simulink model "sim3d_visualization"  (R2024a)
settings: Solver=VariableStepAuto  StartTime=0  StopTime=20  FixedStep=timeStep  RelTol=1e-3
libraries: sim3dlib x4, sim3dautolib x1
settings Model: Creator=The MathWorks, Inc.  LastModifiedBy=nobuakif
settings DataIOCC: SaveOutput=off  DSMLogging=off  InspectSignalLogs=on  SaveTime=off  ReturnWorkspaceOutputs=off
settings OptimizationCC: DefaultParameterBehavior=Inlined  ReuseModelBlockBuffer=off
settings DebuggingCC: ParameterTunabilityLossMsg=error  UnconnectedInputMsg=warning  UnconnectedOutputMsg=warning  UnconnectedLineMsg=warning
settings ModelReferenceCC: EnableRefExpFcnMdlSchedulingChecks=on  PropagateSignalLabelsOutOfModel=off
settings RTWCC: GenCodeOnly=on  GenerateReport=on  GPUComputeCapability=3.5
settings CodeAppCC: ForceParamTrailComments=on
settings GRTTargetCC: TargetLangStandard=C89/C90 (ANSI)

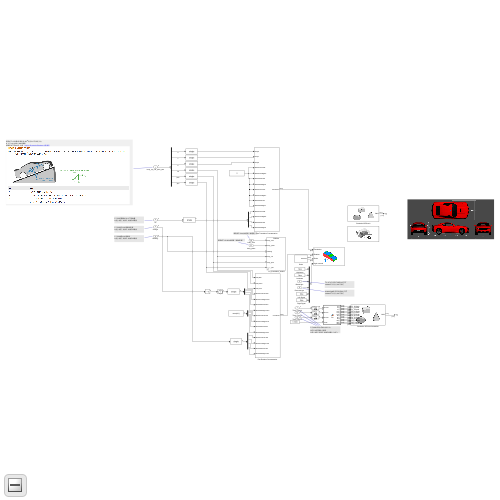
[thumbnail: Simulink's stored preview of the top-level diagram]
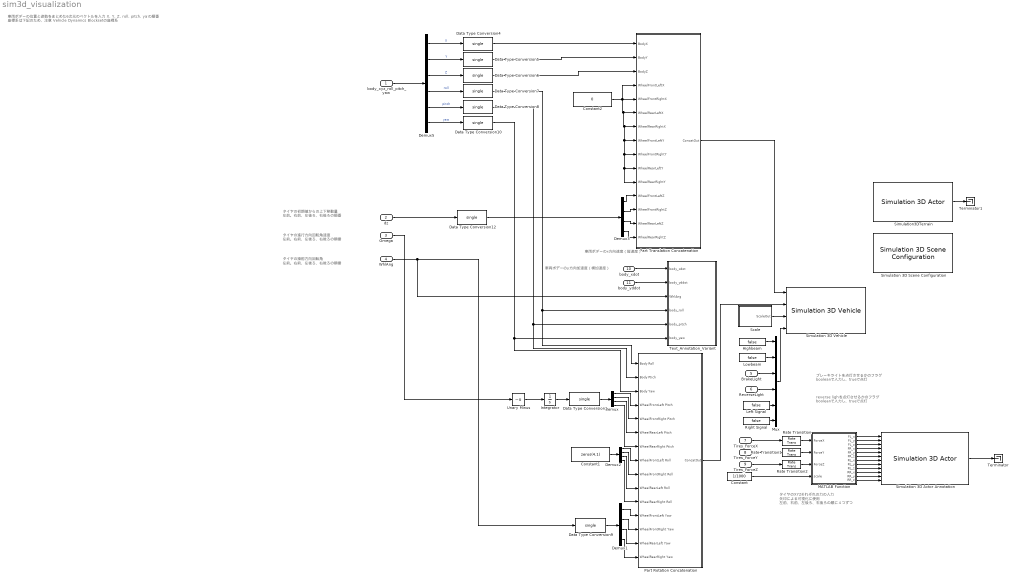
== system sim3d_visualization ==
  note: タイヤの初期値からの上下移動量
      | 左前。右前、左後ろ、右後ろの順番
  note: 車両ボデーの位置と姿勢をまとめた6次元のベクトルを入力
      | X, Y, Z, roll, pitch, yawの順番
      | 座標系は下記のため、注意 Vehicle Dynamics Blockset の座標系
  note: タイヤの進行方向回転角速度
      | 左前。右前、左後ろ、右後ろの順番
  note: タイヤの操舵方向回転角
      | 左前。右前、左後ろ、右後ろの順番
  note: ブレーキライトを点灯させるかのフラグ
      | booleanで入力し、trueで点灯
  note: reverse lightを点灯させるかのフラグ
      | booleanで入力し、trueで点灯
  note: 車両ボデーのx方向速度（縦速度）
  note: 車両ボデーのy方向加速度（横加速度）
  note: タイヤのXYZそれぞれの力の入力
      | 矢印による可視化に使用
      | 左前、右前、左後ろ、右後ろの順に４つずつ
  body_xyz_roll_pitch_yaw : Inport  OutDataTypeStr=single
  dz : Inport  Port=2  OutDataTypeStr=single
  Omega : Inport  Port=3  OutDataTypeStr=double
  WhlAng : Inport  Port=4  OutDataTypeStr=single
  BrakeLight : Inport  Port=5  OutDataTypeStr=boolean
  ReverseLight : Inport  Port=6  OutDataTypeStr=boolean
  Tires_ForceX : Inport  Port=7  OutDataTypeStr=single  PortDimensions=4
  Tires_ForceY : Inport  Port=8  OutDataTypeStr=single  PortDimensions=4
  Tires_ForceZ : Inport  Port=9  OutDataTypeStr=single  PortDimensions=4
  body_xdot : Inport  Port=10  OutDataTypeStr=single
  body_yddot : Inport  Port=11  OutDataTypeStr=single
  Constant : Constant  Value=1/1000
  Constant1 : Constant  Value=zeros(4,1)  OutDataTypeStr=single
  Constant2 : Constant  Value=0  OutDataTypeStr=single
  Data Type Conversion{1,4..10,12} (9 alike) : DataTypeConversion  OutDataTypeStr=single  SaturateOnIntegerOverflow=off  RndMeth=Floor
  Demux{,1..3} (4 alike) : Demux
  Demux5 : Demux  Outputs=6
  Highbeam : Constant  Value=false
  Integrator : Integrator  WrapState=on  WrappedStateUpperValue=2*pi  WrappedStateLowerValue=0  ZeroCross=off
  Left Signal : Constant  Value=false
  Lowbeam : Constant  Value=false
  MATLAB Function : MATLAB Function  TreatAsAtomicUnit=on
  Mux : Mux  Inputs=6
  Part Rotation Concatenation : Subsystem
  Part Translation Concatenation : Subsystem
  Rate Transition : RateTransition  OutPortSampleTime=0.1
  Rate Transition1 : RateTransition  OutPortSampleTime=0.1
  Rate Transition2 : RateTransition  OutPortSampleTime=0.1
  Right Signal : Constant  Value=false
  Scale : Subsystem
  Simulation 3D Actor Annotation : sim3dlib/Simulation 3D Actor  Priority=1  ActorName=Sim3dActor_annotation  ParentName=SimulinkVehicle1  Operation=Create at setup  InitScriptText=|  SampleTime=-1  Translation=single([0 0 0])  Rotation=single([0 0 0])  Scale=single([1 1 1])  InputsText=|  aMode=5  ActorTag=Sim3dActor_annotation  ActorType=Sim3dActor  ID=C
      InitScriptText=|
      | y_offset = 1; z_offset = 0.1;
      | fl_pos = [1.491, 1.713/2+y_offset, z_offset];
      | fr_pos = [1.491, -1.713/2-y_offset, z_offset];
      | rl_pos = [-1.592, 1.713/2+y_offset, z_offset];
      | rr_pos = [-1.592, -1.713/2-y_offset, z_offset];
      | 
      | arrowfl = sim3d.graphics.Arrow("ActorName", "FL_Z");
      | arrowfl.CoordinateSystem = "MATLAB";
      | arrowfl.Color = [0, 0, 1];
      | arrowfl.Rotation = [0, -pi/2, 0];
      | arrowfl.Scale = [1, 1, 1]*2;
      | World.add(arrowfl, Actor);
      | arrowfl.Translation = fl_pos;
      | 
      | arrowfl_x = sim3d.graphics.Arrow("ActorName", "FL_X");
      | arrowfl_x.CoordinateSystem = "MATLAB";
      | arrowfl_x.Color = [1, 0, 0];
      | arrowfl_x.Rotation = [0, 0, 0];
      | arrowfl_x.Scale = [1, 1, 1]*2;
      | World.add(arrowfl_x, Actor);
      | arrowfl_x.Translation = fl_pos;
      | 
      | arrowfl_y = sim3d.graphics.Arrow("ActorName", "FL_Y");
      | arrowfl_y.CoordinateSystem = "MATLAB";
      | arrowfl_y.Color = [0, 1, 0];
      | arrowfl_y.Rotation = [0, 0, pi/2];
      | arrowfl_y.Scale = [1, 1, 1]*2;
      | World.add(arrowfl_y, Actor);
      | arrowfl_y.Translation = fl_pos;
      | 
      | 
      | arrowfr = sim3d.graphics.Arrow("ActorName", "FR_Z");
      | arrowfr.CoordinateSystem = "MATLAB";
      | arrowfr.Color = [0, 0, 1];
      | arrowfr.Rotation = [0, -pi/2, 0];
      | arrowfr.Scale = [1, 1, 1] * 2;
      | World.add(arrowfr, Actor);
      | arrowfr.Translation = fr_pos;
      | 
      | arrowfr_x = sim3d.graphics.Arrow("ActorName", "FR_X");
      | arrowfr_x.CoordinateSystem = "MATLAB";
      | arrowfr_x.Color = [1, 0, 0];
      | arrowfr_x.Rotation = [0, 0, 0];
      | arrowfr_x.Scale = [1, 1, 1]*2;
      | World.add(arrowfr_x, Actor);
      | arrowfr_x.Translation = fr_pos;
      | 
      | arrowfr_y = sim3d.graphics.Arrow("ActorName", "FR_Y");
      | arrowfr_y.CoordinateSystem = "MATLAB";
      | arrowfr_y.Color = [0, 1, 0];
      | arrowfr_y.Rotation = [0, 0, pi/2];
      | arrowfr_y.Scale = [1, 1, 1]*2;
      | World.add(arrowfr_y, Actor);
      | arrowfr_y.Translation = fr_pos;
      | 
      | 
      | arrowrl = sim3d.graphics.Arrow("ActorName", "RL_Z");
      | arrowrl.CoordinateSystem = "MATLAB";
      | arrowrl.Color = [0, 0, 1];
      | arrowrl.Rotation = [0, -pi/2, 0];
      | arrowrl.Scale = [1, 1, 1] * 2;
      | World.add(arrowrl, Actor);
      | arrowrl.Translation = rl_pos;
      | 
      | arrowrl_x = sim3d.graphics.Arrow("ActorName", "RL_X");
      | arrowrl_x.CoordinateSystem = "MATLAB";
      | arrowrl_x.Color = [1, 0, 0];
      | arrowrl_x.Rotation = [0, 0, 0];
      | arrowrl_x.Scale = [1, 1, 1]*2;
      | World.add(arrowrl_x, Actor);
      | arrowrl_x.Translation = rl_pos;
      | 
      | arrowrl_y = sim3d.graphics.Arrow("ActorName", "RL_Y");
      | arrowrl_y.CoordinateSystem = "MATLAB";
      | arrowrl_y.Color = [0, 1, 0];
      | arrowrl_y.Rotation = [0, 0, pi/2];
      | arrowrl_y.Scale = [1, 1, 1]*2;
      | World.add(arrowrl_y, Actor);
      | arrowrl_y.Translation = rl_pos;
      | 
      | 
      | arrowrr = sim3d.graphics.Arrow("ActorName", "RR_Z");
      | arrowrr.CoordinateSystem = "MATLAB";
      | arrowrr.Color = [0, 0, 1];
      | arrowrr.Rotation = [0, -pi/2, 0];
      | arrowrr.Scale = [1, 1, 1]*2;
      | World.add(arrowrr, Actor);
      | arrowrr.Translation = rr_pos;
      | 
      | arrowrr_x = sim3d.graphics.Arrow("ActorName", "RR_X");
      | arrowrr_x.CoordinateSystem = "MATLAB";
      | arrowrr_x.Color = [1, 0, 0];
      | arrowrr_x.Rotation = [0, 0, 0];
      | arrowrr_x.Scale = [1, 1, 1]*2;
      | World.add(arrowrr_x, Actor);
      | arrowrr_x.Translation = rr_pos;
      | 
      | arrowrr_y = sim3d.graphics.Arrow("ActorName", "RR_Y");
      | arrowrr_y.CoordinateSystem = "MATLAB";
      | arrowrr_y.Color = [0, 1, 0];
      | arrowrr_y.Rotation = [0, 0, pi/2];
      | arrowrr_y.Scale = [1, 1, 1]*2;
      | World.add(arrowrr_y, Actor);
      | arrowrr_y.Translation = rr_pos;
      InputsText=|
      | FL_X.Scale
      | FL_Y.Scale
      | FL_Z.Scale
      | FR_X.Scale
      | FR_Y.Scale
      | FR_Z.Scale
      | RL_X.Scale
      | RL_Y.Scale
      | RL_Z.Scale
      | RR_X.Scale
      | RR_Y.Scale
      | RR_Z.Scale
  Simulation 3D Scene Configuration : sim3dlib/Simulation 3D Scene Configuration  Priority=0  ProjectFormat=Default Scenes  SceneDesc=Empty scene  ProjectName=D:\MATLAB\R2024a\toolbox\shared\sim3d_projects\automotive_project_windows\UE\WindowsNoEditor\VehicleSimulation.exe  ScenePath=/Game/Maps/HwStrght  RoadRunnerProjectPath=D:\MATLAB\RoadRunnerSimulinkHandson_github\CRG\crgRoad.stl  EnableOpenDRIVE=off  vehTagList={'Custom';'Scene Origin';'Sim3dActor1';'Sim3dActor_annotation';'Sim3dActor_text';'SimulinkVehicle1'}  vehTag=SimulinkVehicle1  FreeCameraInitialTranslation=[0, 0, 0]  FreeCameraDefaultInitialTranslation=[-6, 0, 2]  FreeCameraInitialRotation=[0, 0, 0]  FreeCameraDefaultInitialRotation=[0, -15, 0]  OpVisEn=off  Ts=0.1  EnableWindow=on  EnableRemoteAccess=off  EnableWeather=off  SunAzimuth=90  SunAltitude=40.0  EnableGeospatialSun=off  Latitude=0  Longitude=0  Date=2023-01-01  Time=10:30:00  GeoTimeZone=-5.0  SunDaylightSaving=off  wind=1  clouds=10  EnableVolumetricClouds=off  CloudCoverage=0  CloudAltitude=6  fog=0  rain=0  RaindropsEffect=off  SnowDensity=0  EnableGeospatial=off  UseTrueOrigin=off  OriginHeight=200  OriginLatitude=40.744652  OriginLongitude=-73.988864  MapStyle=Aerial  AdditionalAssetIDs=[]  UseAdvancedSunSky=off  SolarTime=11  TimeZone=-5  Day=21  Month=9  Year=2022  UseDaylightSavingTime=on  DSTStartDay=10  DSTStartMonth=3  DSTEndDay=3  DSTEndMonth=11  DSTSwitchHour=2  sensorTag=MainCamera1  sensorId=1  sensorName=MainCamera1  mountLoc=Origin  offsetFlag=off  tmountOffset=[0, 0, 0]  rmountOffset=[0, 0, 0]  HorizontalResolution=1280  VerticalResolution=720  HorizontalFOV=60  mountPoint=[0 0 0]  mountOrientation=[0 0 0]  aMode=5  ID=1  GeoTrigger=Inactive
      settings: LibrarySourceBlock=sl3dlib/Simulation 3D/Simulation 3D Scene Configuration
  Simulation 3D Vehicle : sim3dautolib/Simulation 3D Vehicle  Priority=-1  PassVehMesh=Muscle car  MeshPath=/MathWorksSimulation/Vehicles/Muscle/Meshes/SK_MuscleCar.SK_MuscleCar  VehColor=Red  ActorName=SimulinkVehicle1  VehLightsControl=on  HeadlightColor=[ 1, 1, 1 ]  HighBeamIntensity=100000  LowBeamIntensity=60000  HighBeamConeAngle=1.22  LowBeamConeAngle=1.22  LeftHeadlightOrientation=[ 0, 0 ]  RightHeadlightOrientation=[ 0, 0 ]  BrakelightIntensity=500  ReverselightIntensity=500  SignallightIntensity=500  SignallightPeriod=1  SignalPulseWidth=50  Translation=zeros(5,3)  Rotation=zeros(5,3)  Scale=ones( 5, 3 )  SampleTime=-1  ActorType=SimulinkVehicle  ID=1  aMode=2  ActorTag=SimulinkVehicle1
  Simulation3DTerrain : sim3dlib/Simulation 3D Actor  Priority=1  ActorName=Sim3dActor1  ParentName=Scene Origin  Operation=Create at setup  InitScriptText="Actor.CoordinateSystem = \"MATLAB\";"  SampleTime=-1  Translation=[0 0 0]  Rotation=[0 0 0]  Scale=[1 1 1]  aMode=5  ActorTag=Sim3dActor1  ActorType=Sim3dActor  ID=1
  Terminator : Terminator
  Terminator1 : Terminator
  Text_Annotation_Variant : Subsystem  Priority=1  Variant=on
  Unary Minus : UnaryMinus
  wires:
  Demux5/6 -> Data Type Conversion10/1  "yaw"
  Demux5/3 -> Data Type Conversion6/1  "Z"
  MATLAB Function/5(FR_y) -> Simulation 3D Actor Annotation/5
  MATLAB Function/8(RL_y) -> Simulation 3D Actor Annotation/8
  Right Signal/1 -> Mux/6
  Demux3/2 -> Part Translation Concatenation/13(WheelFrontRightZ)
  MATLAB Function/9(RL_z) -> Simulation 3D Actor Annotation/9
  Mux/1 -> Simulation 3D Vehicle/4
  Constant1/1 -> Demux2/1
  Data Type Conversion6/1 -> Part Translation Concatenation/3(BodyZ)
  MATLAB Function/1(FL_x) -> Simulation 3D Actor Annotation/1
  Omega/1 -> Unary Minus/1
  Part Translation Concatenation/1(ConcatOut) -> Simulation 3D Vehicle/1
  MATLAB Function/11(RR_y) -> Simulation 3D Actor Annotation/11
  MATLAB Function/7(RL_x) -> Simulation 3D Actor Annotation/7
  Demux3/3 -> Part Translation Concatenation/14(WheelRearLeftZ)
  Demux5/4 -> Data Type Conversion7/1  "roll"
  MATLAB Function/2(FL_y) -> Simulation 3D Actor Annotation/2
  Demux1/2 -> Part Rotation Concatenation/13(WheelFrontRight Yaw)
  Demux3/1 -> Part Translation Concatenation/12(WheelFrontLeftZ)
  Demux2/1 -> Part Rotation Concatenation/8(WheelFrontLeft Roll)
  Demux2/3 -> Part Rotation Concatenation/10(WheelRearLeft Roll)
  Tires_ForceY/1 -> Rate Transition1/1
  Tires_ForceX/1 -> Rate Transition/1
  Unary Minus/1 -> Integrator/1
  Lowbeam/1 -> Mux/2
  MATLAB Function/6(FR_z) -> Simulation 3D Actor Annotation/6
  MATLAB Function/10(RR_x) -> Simulation 3D Actor Annotation/10
  MATLAB Function/4(FR_x) -> Simulation 3D Actor Annotation/4
  Constant2/1 -> Part Translation Concatenation/5(WheelFrontRightX), Part Translation Concatenation/6(WheelRearLeftX), Part Translation Concatenation/7(WheelRearRightX), Part Translation Concatenation/8(WheelFrontLeftY), Part Translation Concatenation/9(WheelFrontRightY), Part Translation Concatenation/10(WheelRearLeftY), Part Translation Concatenation/11(WheelRearRightY), Part Translation Concatenation/4(WheelFrontLeftX)
  BrakeLight/1 -> Mux/3
  Part Rotation Concatenation/1(ConcatOut) -> Simulation 3D Vehicle/2
  Data Type Conversion7/1 -> Text_Annotation_Variant/4(body_roll), Part Rotation Concatenation/1(Body Roll)
  MATLAB Function/3(FL_z) -> Simulation 3D Actor Annotation/3
  Integrator/1 -> Data Type Conversion1/1
  Demux5/5 -> Data Type Conversion8/1  "pitch"
  Simulation 3D Actor Annotation/1 -> Terminator/1
  Data Type Conversion4/1 -> Part Translation Concatenation/1(BodyX)
  Left Signal/1 -> Mux/5
  Demux5/1 -> Data Type Conversion4/1  "X"
  Demux/3 -> Part Rotation Concatenation/6(WheelRearLeft Pitch)
  Demux5/2 -> Data Type Conversion5/1  "Y"
  Data Type Conversion12/1 -> Demux3/1
  Demux1/4 -> Part Rotation Concatenation/15(WheelRearRight Yaw)
  Data Type Conversion8/1 -> Part Rotation Concatenation/2(Body Ptich), Text_Annotation_Variant/5(body_pitch)
  ReverseLight/1 -> Mux/4
  Demux1/1 -> Part Rotation Concatenation/12(WheelFrontLeft Yaw)
  Tires_ForceZ/1 -> Rate Transition2/1
  Data Type Conversion9/1 -> Demux1/1
  MATLAB Function/12(RR_z) -> Simulation 3D Actor Annotation/12
  Data Type Conversion10/1 -> Part Rotation Concatenation/3(Body Yaw), Text_Annotation_Variant/6(body_yaw)
  Scale/1(ScaleOut) -> Simulation 3D Vehicle/3
  Demux/1 -> Part Rotation Concatenation/4(WheelFrontLeft Pitch)
  Highbeam/1 -> Mux/1
  Demux3/4 -> Part Translation Concatenation/15(WheelRearRightZ)
  WhlAng/1 -> Text_Annotation_Variant/3(WhlAng), Data Type Conversion9/1
  dz/1 -> Data Type Conversion12/1
  Demux/2 -> Part Rotation Concatenation/5(WheelFrontRight Pitch)
  Demux2/4 -> Part Rotation Concatenation/11(WheelRearRight Roll)
  Demux2/2 -> Part Rotation Concatenation/9(WheelFrontRight Roll)
  Data Type Conversion5/1 -> Part Translation Concatenation/2(BodyY)
  Demux/4 -> Part Rotation Concatenation/7(WheelRearRight Ptich)
  Demux1/3 -> Part Rotation Concatenation/14(WheelRearLeft Yaw)
  body_xyz_roll_pitch_yaw/1 -> Demux5/1
  body_xdot/1 -> Text_Annotation_Variant/1(body_xdot)
  body_yddot/1 -> Text_Annotation_Variant/2(body_yddot)
  Constant/1 -> MATLAB Function/4(scale)
  Data Type Conversion1/1 -> Demux/1
  Simulation3DTerrain/1 -> Terminator1/1
  Rate Transition/1 -> MATLAB Function/1(ForceX)
  Rate Transition1/1 -> MATLAB Function/2(ForceY)
  Rate Transition2/1 -> MATLAB Function/3(ForceZ)

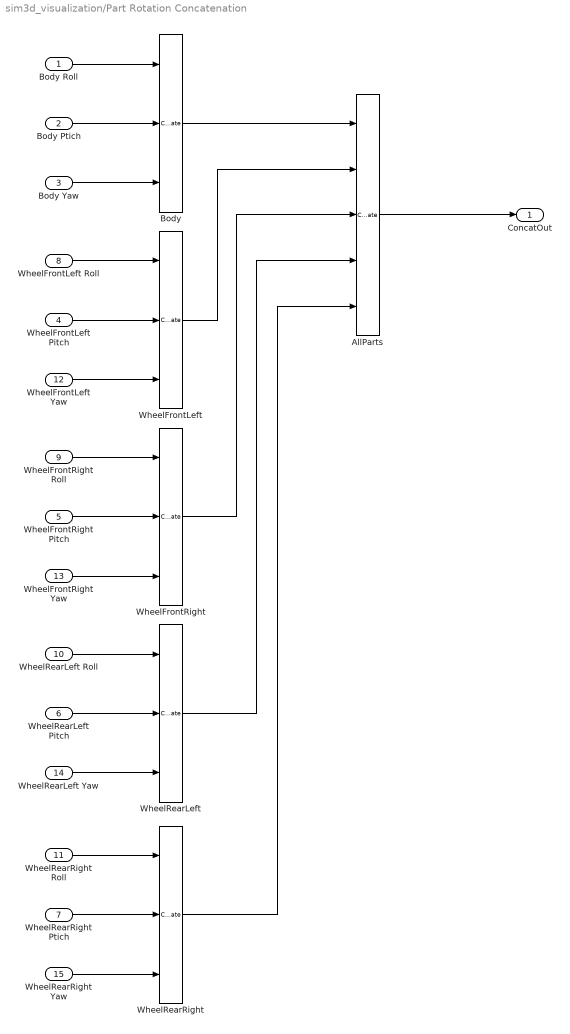
== system sim3d_visualization/Part Rotation Concatenation ==
  Body Roll : Inport
  Body Ptich : Inport  Port=2
  Body Yaw : Inport  Port=3
  WheelFrontLeft Pitch : Inport  Port=4
  WheelFrontRight Pitch : Inport  Port=5
  WheelRearLeft Pitch : Inport  Port=6
  WheelRearRight Ptich : Inport  Port=7
  WheelFrontLeft Roll : Inport  Port=8
  WheelFrontRight Roll : Inport  Port=9
  WheelRearLeft Roll : Inport  Port=10
  WheelRearRight Roll : Inport  Port=11
  WheelFrontLeft Yaw : Inport  Port=12
  WheelFrontRight Yaw : Inport  Port=13
  WheelRearLeft Yaw : Inport  Port=14
  WheelRearRight Yaw : Inport  Port=15
  AllParts : Concatenate  NumInputs=5  Mode=Multidimensional array
  Body : Concatenate  NumInputs=3  Mode=Multidimensional array  ConcatenateDimension=2
  WheelFrontLeft : Concatenate  NumInputs=3  Mode=Multidimensional array  ConcatenateDimension=2
  WheelFrontRight : Concatenate  NumInputs=3  Mode=Multidimensional array  ConcatenateDimension=2
  WheelRearLeft : Concatenate  NumInputs=3  Mode=Multidimensional array  ConcatenateDimension=2
  WheelRearRight : Concatenate  NumInputs=3  Mode=Multidimensional array  ConcatenateDimension=2
  ConcatOut : Outport  VectorParamsAs1DForOutWhenUnconnected=off
  wires:
  Body Yaw/1 -> Body/3
  WheelFrontLeft Yaw/1 -> WheelFrontLeft/3
  WheelFrontLeft/1 -> AllParts/2
  Body/1 -> AllParts/1
  WheelRearLeft/1 -> AllParts/4
  WheelFrontRight/1 -> AllParts/3
  WheelRearRight Yaw/1 -> WheelRearRight/3
  WheelRearLeft Yaw/1 -> WheelRearLeft/3
  AllParts/1 -> ConcatOut/1
  WheelRearRight/1 -> AllParts/5
  WheelFrontRight Yaw/1 -> WheelFrontRight/3
  Body Roll/1 -> Body/1
  Body Ptich/1 -> Body/2
  WheelFrontLeft Pitch/1 -> WheelFrontLeft/2
  WheelFrontLeft Roll/1 -> WheelFrontLeft/1
  WheelFrontRight Roll/1 -> WheelFrontRight/1
  WheelFrontRight Pitch/1 -> WheelFrontRight/2
  WheelRearLeft Roll/1 -> WheelRearLeft/1
  WheelRearLeft Pitch/1 -> WheelRearLeft/2
  WheelRearRight Roll/1 -> WheelRearRight/1
  WheelRearRight Ptich/1 -> WheelRearRight/2

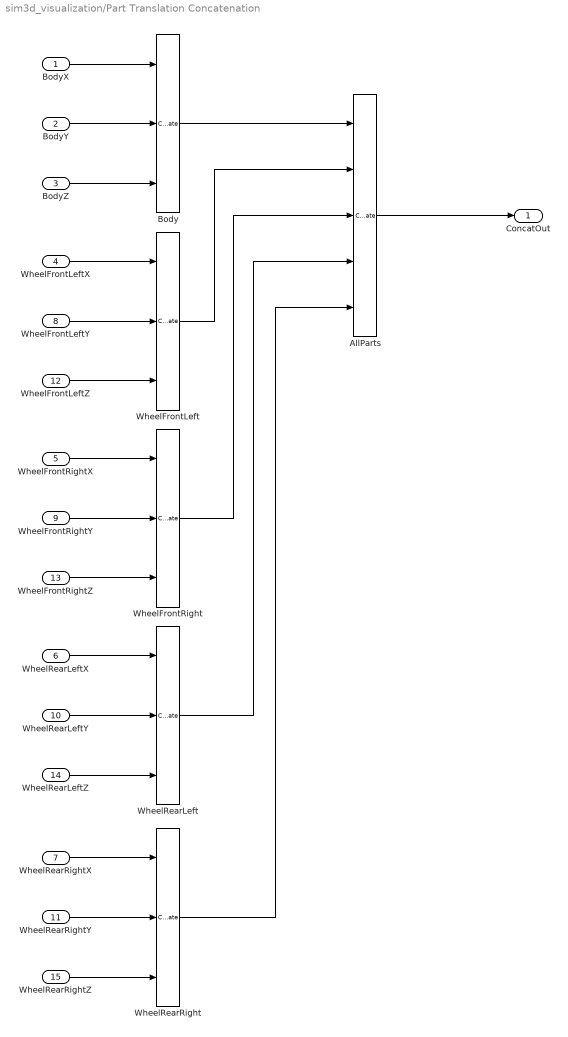
== system sim3d_visualization/Part Translation Concatenation ==
  BodyX : Inport
  BodyY : Inport  Port=2
  BodyZ : Inport  Port=3
  WheelFrontLeftX : Inport  Port=4
  WheelFrontRightX : Inport  Port=5
  WheelRearLeftX : Inport  Port=6
  WheelRearRightX : Inport  Port=7
  WheelFrontLeftY : Inport  Port=8
  WheelFrontRightY : Inport  Port=9
  WheelRearLeftY : Inport  Port=10
  WheelRearRightY : Inport  Port=11
  WheelFrontLeftZ : Inport  Port=12
  WheelFrontRightZ : Inport  Port=13
  WheelRearLeftZ : Inport  Port=14
  WheelRearRightZ : Inport  Port=15
  AllParts : Concatenate  NumInputs=5  Mode=Multidimensional array
  Body : Concatenate  NumInputs=3  Mode=Multidimensional array  ConcatenateDimension=2
  WheelFrontLeft : Concatenate  NumInputs=3  Mode=Multidimensional array  ConcatenateDimension=2
  WheelFrontRight : Concatenate  NumInputs=3  Mode=Multidimensional array  ConcatenateDimension=2
  WheelRearLeft : Concatenate  NumInputs=3  Mode=Multidimensional array  ConcatenateDimension=2
  WheelRearRight : Concatenate  NumInputs=3  Mode=Multidimensional array  ConcatenateDimension=2
  ConcatOut : Outport  VectorParamsAs1DForOutWhenUnconnected=off
  wires:
  BodyX/1 -> Body/1
  BodyZ/1 -> Body/3
  WheelFrontLeftX/1 -> WheelFrontLeft/1
  WheelFrontLeftZ/1 -> WheelFrontLeft/3
  WheelFrontLeftY/1 -> WheelFrontLeft/2
  BodyY/1 -> Body/2
  WheelFrontLeft/1 -> AllParts/2
  WheelRearRightX/1 -> WheelRearRight/1
  Body/1 -> AllParts/1
  WheelRearLeft/1 -> AllParts/4
  WheelFrontRight/1 -> AllParts/3
  WheelRearRightZ/1 -> WheelRearRight/3
  WheelFrontRightY/1 -> WheelFrontRight/2
  WheelFrontRightX/1 -> WheelFrontRight/1
  WheelRearRightY/1 -> WheelRearRight/2
  WheelRearLeftZ/1 -> WheelRearLeft/3
  AllParts/1 -> ConcatOut/1
  WheelRearLeftY/1 -> WheelRearLeft/2
  WheelRearRight/1 -> AllParts/5
  WheelRearLeftX/1 -> WheelRearLeft/1
  WheelFrontRightZ/1 -> WheelFrontRight/3

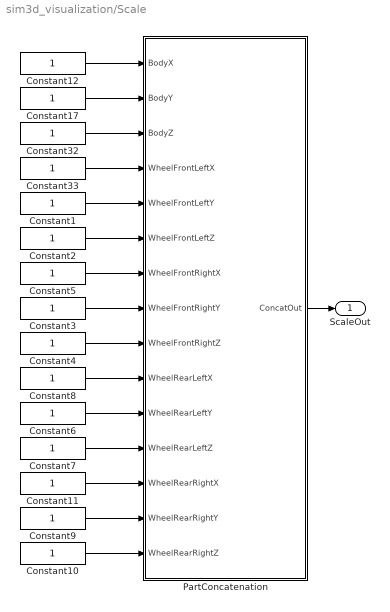
== system sim3d_visualization/Scale ==
  Constant{1..12,17,32..33} (15 alike) : Constant  OutDataTypeStr=single
  PartConcatenation : Subsystem
  ScaleOut : Outport  VectorParamsAs1DForOutWhenUnconnected=off
  wires:
  Constant10/1 -> PartConcatenation/15(WheelRearRightZ)
  Constant9/1 -> PartConcatenation/14(WheelRearRightY)
  Constant11/1 -> PartConcatenation/13(WheelRearRightX)
  Constant7/1 -> PartConcatenation/12(WheelRearLeftZ)
  Constant6/1 -> PartConcatenation/11(WheelRearLeftY)
  Constant8/1 -> PartConcatenation/10(WheelRearLeftX)
  Constant4/1 -> PartConcatenation/9(WheelFrontRightZ)
  Constant3/1 -> PartConcatenation/8(WheelFrontRightY)
  Constant5/1 -> PartConcatenation/7(WheelFrontRightX)
  Constant2/1 -> PartConcatenation/6(WheelFrontLeftZ)
  Constant1/1 -> PartConcatenation/5(WheelFrontLeftY)
  Constant33/1 -> PartConcatenation/4(WheelFrontLeftX)
  Constant32/1 -> PartConcatenation/3(BodyZ)
  Constant17/1 -> PartConcatenation/2(BodyY)
  Constant12/1 -> PartConcatenation/1(BodyX)
  PartConcatenation/1(ConcatOut) -> ScaleOut/1

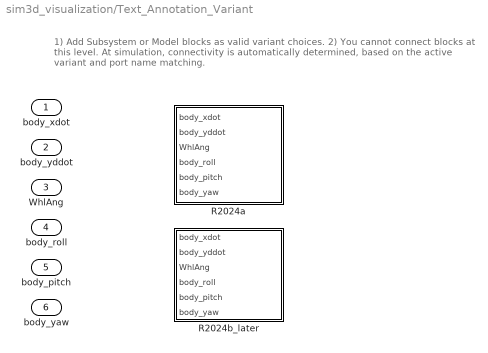
== system sim3d_visualization/Text_Annotation_Variant ==
  note: 1) Add Subsystem or Model blocks as valid variant choices.
      | 2) You cannot connect blocks at this level. At simulation, connectivity is automatically
      | determined, based on the active variant and port name matching.
  body_xdot : Inport
  body_yddot : Inport  Port=2
  WhlAng : Inport  Port=3
  body_roll : Inport  Port=4
  body_pitch : Inport  Port=5
  body_yaw : Inport  Port=6
  R2024a : Subsystem  VariantControl=str2num(ver('simulink').Version) <= 24.1
  R2024b_later : Subsystem  VariantControl=str2num(ver('simulink').Version) > 24.1

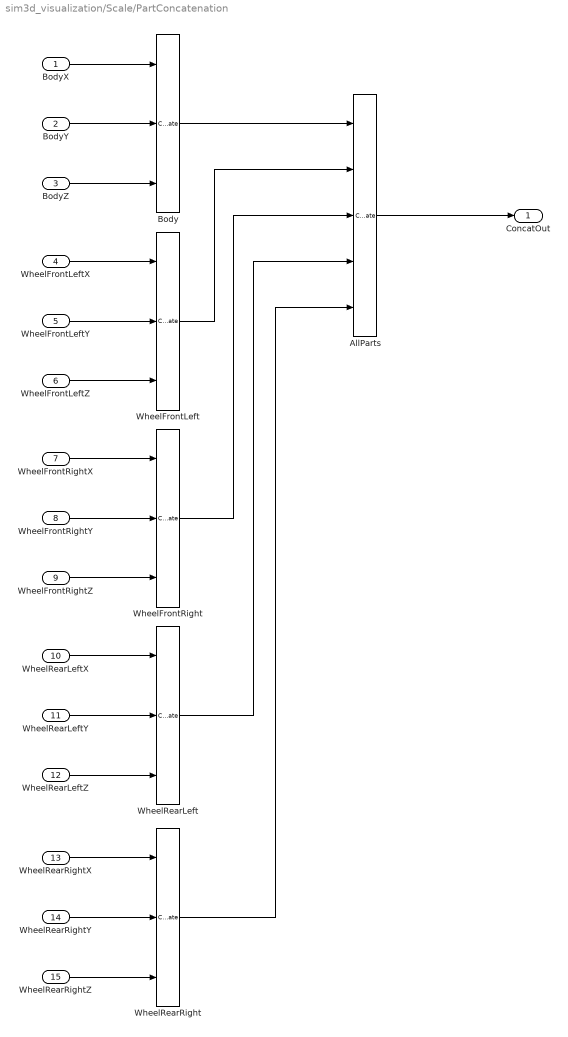
== system sim3d_visualization/Scale/PartConcatenation ==
  BodyX : Inport
  BodyY : Inport  Port=2
  BodyZ : Inport  Port=3
  WheelFrontLeftX : Inport  Port=4
  WheelFrontLeftY : Inport  Port=5
  WheelFrontLeftZ : Inport  Port=6
  WheelFrontRightX : Inport  Port=7
  WheelFrontRightY : Inport  Port=8
  WheelFrontRightZ : Inport  Port=9
  WheelRearLeftX : Inport  Port=10
  WheelRearLeftY : Inport  Port=11
  WheelRearLeftZ : Inport  Port=12
  WheelRearRightX : Inport  Port=13
  WheelRearRightY : Inport  Port=14
  WheelRearRightZ : Inport  Port=15
  AllParts : Concatenate  NumInputs=5  Mode=Multidimensional array
  Body : Concatenate  NumInputs=3  Mode=Multidimensional array  ConcatenateDimension=2
  WheelFrontLeft : Concatenate  NumInputs=3  Mode=Multidimensional array  ConcatenateDimension=2
  WheelFrontRight : Concatenate  NumInputs=3  Mode=Multidimensional array  ConcatenateDimension=2
  WheelRearLeft : Concatenate  NumInputs=3  Mode=Multidimensional array  ConcatenateDimension=2
  WheelRearRight : Concatenate  NumInputs=3  Mode=Multidimensional array  ConcatenateDimension=2
  ConcatOut : Outport  VectorParamsAs1DForOutWhenUnconnected=off
  wires:
  BodyX/1 -> Body/1
  BodyZ/1 -> Body/3
  WheelFrontLeftX/1 -> WheelFrontLeft/1
  WheelFrontLeftZ/1 -> WheelFrontLeft/3
  WheelFrontLeftY/1 -> WheelFrontLeft/2
  BodyY/1 -> Body/2
  WheelFrontLeft/1 -> AllParts/2
  WheelRearRightX/1 -> WheelRearRight/1
  Body/1 -> AllParts/1
  WheelRearLeft/1 -> AllParts/4
  WheelFrontRight/1 -> AllParts/3
  WheelRearRightZ/1 -> WheelRearRight/3
  WheelFrontRightY/1 -> WheelFrontRight/2
  WheelFrontRightX/1 -> WheelFrontRight/1
  WheelRearRightY/1 -> WheelRearRight/2
  WheelRearLeftZ/1 -> WheelRearLeft/3
  AllParts/1 -> ConcatOut/1
  WheelRearLeftY/1 -> WheelRearLeft/2
  WheelRearRight/1 -> AllParts/5
  WheelRearLeftX/1 -> WheelRearLeft/1
  WheelFrontRightZ/1 -> WheelFrontRight/3

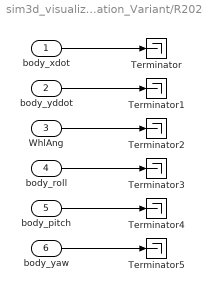
== system sim3d_visualization/Text_Annotation_Variant/R2024a ==
  body_xdot : Inport
  body_yddot : Inport  Port=2
  WhlAng : Inport  Port=3
  body_roll : Inport  Port=4
  body_pitch : Inport  Port=5
  body_yaw : Inport  Port=6
  Terminator{,1..5} (6 alike) : Terminator
  wires:
  body_xdot/1 -> Terminator/1
  body_yddot/1 -> Terminator1/1
  WhlAng/1 -> Terminator2/1
  body_roll/1 -> Terminator3/1
  body_pitch/1 -> Terminator4/1
  body_yaw/1 -> Terminator5/1

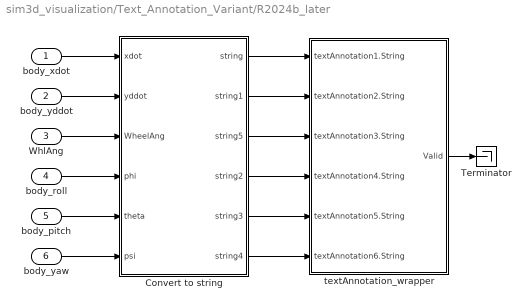
== system sim3d_visualization/Text_Annotation_Variant/R2024b_later ==
  body_xdot : Inport
  body_yddot : Inport  Port=2
  WhlAng : Inport  Port=3
  body_roll : Inport  Port=4
  body_pitch : Inport  Port=5
  body_yaw : Inport  Port=6
  Convert to string : Subsystem
  Terminator : Terminator
  textAnnotation_wrapper : Subsystem  Priority=1  Variant=on  AllowZeroVariantControls=on
  wires:
  Convert to string/5(string3) -> textAnnotation_wrapper/5(textAnnotation5.String)
  Convert to string/2(string1) -> textAnnotation_wrapper/2(textAnnotation2.String)
  Convert to string/4(string2) -> textAnnotation_wrapper/4(textAnnotation4.String)
  Convert to string/6(string4) -> textAnnotation_wrapper/6(textAnnotation6.String)
  Convert to string/3(string5) -> textAnnotation_wrapper/3(textAnnotation3.String)
  body_pitch/1 -> Convert to string/5(theta)
  body_yaw/1 -> Convert to string/6(psi)
  WhlAng/1 -> Convert to string/3(WheelAng)
  body_yddot/1 -> Convert to string/2(yddot)
  body_roll/1 -> Convert to string/4(phi)
  body_xdot/1 -> Convert to string/1(xdot)
  Convert to string/1(string) -> textAnnotation_wrapper/1(textAnnotation1.String)
  textAnnotation_wrapper/1(Valid) -> Terminator/1

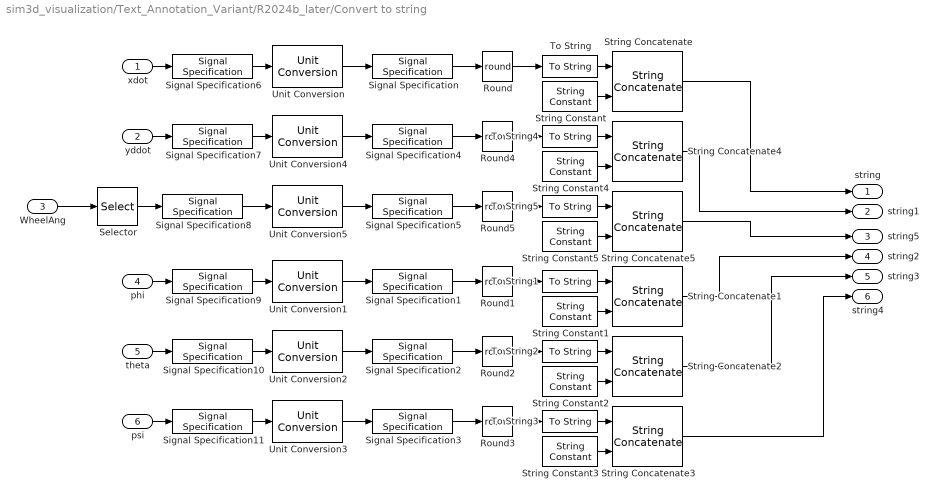
== system sim3d_visualization/Text_Annotation_Variant/R2024b_later/Convert to string ==
  xdot : Inport
  yddot : Inport  Port=2
  WheelAng : Inport  Port=3
  phi : Inport  Port=4
  theta : Inport  Port=5
  psi : Inport  Port=6
  Round{,1..5} (6 alike) : Rounding  Operator=round
  Selector : Selector  InputPortWidth=4  IndexOptions=Index vector (dialog)  Indices=[1]  OutputSizes=1
  Signal Specification : SignalSpecification  Unit=km/h
  Signal Specification{1..3,5} (4 alike) : SignalSpecification  Unit=deg
  Signal Specification{8..11} (4 alike) : SignalSpecification  Unit=rad
  Signal Specification4 : SignalSpecification  Unit=m/s^2
  Signal Specification6 : SignalSpecification  Unit=m/s
  Signal Specification7 : SignalSpecification  Unit=m/s^2
  String Concatenate{,1..5} (6 alike) : StringConcatenate
  String Constant : StringConstant  String="\" km/h\""
  String Constant{1..3,5} (4 alike) : StringConstant  String="\" deg\""
  String Constant4 : StringConstant  String="\" m/s^2\""
  To String{,1..5} (6 alike) : ToString
  Unit Conversion{,1..5} (6 alike) : UnitConversion
  string : Outport
  string1 : Outport  Port=2
  string5 : Outport  Port=3
  string2 : Outport  Port=4
  string3 : Outport  Port=5
  string4 : Outport  Port=6
  wires:
  Selector/1 -> Signal Specification8/1
  String Concatenate5/1 -> string5/1
  WheelAng/1 -> Selector/1
  String Constant5/1 -> String Concatenate5/2
  To String5/1 -> String Concatenate5/1
  Signal Specification5/1 -> Round5/1
  Round5/1 -> To String5/1
  Unit Conversion5/1 -> Signal Specification5/1
  String Concatenate4/1 -> string1/1
  yddot/1 -> Signal Specification7/1
  Unit Conversion4/1 -> Signal Specification4/1
  Round4/1 -> To String4/1
  Signal Specification4/1 -> Round4/1
  To String4/1 -> String Concatenate4/1
  String Constant4/1 -> String Concatenate4/2
  String Concatenate3/1 -> string4/1
  String Concatenate2/1 -> string3/1
  String Concatenate1/1 -> string2/1
  String Concatenate/1 -> string/1
  theta/1 -> Signal Specification10/1
  psi/1 -> Signal Specification11/1
  Unit Conversion3/1 -> Signal Specification3/1
  Round3/1 -> To String3/1
  Signal Specification3/1 -> Round3/1
  To String3/1 -> String Concatenate3/1
  String Constant3/1 -> String Concatenate3/2
  String Constant2/1 -> String Concatenate2/2
  To String2/1 -> String Concatenate2/1
  Signal Specification2/1 -> Round2/1
  Round2/1 -> To String2/1
  Unit Conversion2/1 -> Signal Specification2/1
  phi/1 -> Signal Specification9/1
  Unit Conversion1/1 -> Signal Specification1/1
  Round1/1 -> To String1/1
  Signal Specification1/1 -> Round1/1
  To String1/1 -> String Concatenate1/1
  String Constant1/1 -> String Concatenate1/2
  String Constant/1 -> String Concatenate/2
  To String/1 -> String Concatenate/1
  Signal Specification/1 -> Round/1
  Round/1 -> To String/1
  Unit Conversion/1 -> Signal Specification/1
  xdot/1 -> Signal Specification6/1
  Signal Specification6/1 -> Unit Conversion/1
  Signal Specification7/1 -> Unit Conversion4/1
  Signal Specification8/1 -> Unit Conversion5/1
  Signal Specification9/1 -> Unit Conversion1/1
  Signal Specification10/1 -> Unit Conversion2/1
  Signal Specification11/1 -> Unit Conversion3/1

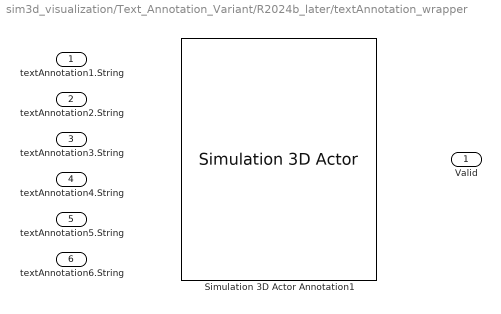
== system sim3d_visualization/Text_Annotation_Variant/R2024b_later/textAnnotation_wrapper ==
  textAnnotation1.String : Inport
  textAnnotation2.String : Inport  Port=2
  textAnnotation3.String : Inport  Port=3
  textAnnotation4.String : Inport  Port=4
  textAnnotation5.String : Inport  Port=5
  textAnnotation6.String : Inport  Port=6
  Simulation 3D Actor Annotation1 : sim3dlib/Simulation 3D Actor  Priority=1  VariantControl=true  ActorName=Sim3dActor_text  ParentName=SimulinkVehicle1  Operation=Create at setup  InitScriptText=|  SampleTime=-1  Translation=single([0 0 0])  Rotation=single([0 0 0])  Scale=single([1 1 1])  InputsText=|  aMode=5  ActorTag=Sim3dActor_text  ActorType=Sim3dActor  ID=C
      InitScriptText=|
      | prefix = ["0 km/h"; "0 m/s^2"; "steer 0 deg"; "Roll 0 deg"; "Pitch 0 deg"; "Yaw 0 deg"];
      | positions = [0, 2, 3; 0, 0, 3; 0, -3, 3;
      |     0, 2, 2; 0, 0, 2; 0, -2, 2];
      | 
      | for i = 1:size(positions, 1)
      | text = sim3d.graphics.Text("ActorName", "textAnnotation"+string(i));
      | text.CoordinateSystem = "MATLAB";
      | text.Translation = positions(i,:);
      | text.String = prefix(i);
      | text.FontSize = 2;
      | add(World, text, actor);
      | end
      InputsText=|
      | textAnnotation1.String
      | textAnnotation2.String
      | textAnnotation3.String
      | textAnnotation4.String
      | textAnnotation5.String
      | textAnnotation6.String
  Valid : Outport

== matlab function sim3d_visualization/MATLAB Function ==
  data: ForceX input; FL_x output; FL_y output; FL_z output; ForceY input; FR_x output; FR_y output; FR_z output; RL_x output; RL_y output; RL_z output; RR_x output; RR_y output; RR_z output; ForceZ input; scale input
function [FL_x, FL_y, FL_z, FR_x, FR_y, FR_z,...
    RL_x, RL_y, RL_z, RR_x, RR_y, RR_z] = fcn(ForceX, ForceY, ForceZ, scale)

FL_x = [ForceX(1)*scale, 2, 2];
FL_y = [ForceY(1)*scale, 2, 2];
FL_z = [ForceZ(1)*scale, 2, 2];

FR_x = [ForceX(2)*scale, 2, 2];
FR_y = [ForceY(2)*scale, 2, 2];
FR_z = [ForceZ(2)*scale, 2, 2];

RL_x = [ForceX(3)*scale, 2, 2];
RL_y = [ForceY(3)*scale, 2, 2];
RL_z = [ForceZ(3)*scale, 2, 2];

RR_x = [ForceX(4)*scale, 2, 2];
RR_y = [ForceY(4)*scale, 2, 2];
RR_z = [ForceZ(4)*scale, 2, 2];
